simulink model "INFLW_2"  (R2022b)
settings: Solver=FixedStepDiscrete  StartTime=0  StopTime=duration  FixedStep=sample_time  RelTol=1e-3
values from neighbouring files (symbols this model uses):
  ParInflow =     [INFLW_2_params.mat]
  sample_time = 0.1    [INFLW_2_params.mat]
libraries: simulink x15, dspstat3 x11
settings Model: Creator=Carlo_TUM  LastModifiedBy=Carlo_TUM
settings DataIOCC: LoadExternalInput=on  ReturnWorkspaceOutputs=off  ReturnWorkspaceOutputsName=off
settings OptimizationCC: DefaultParameterBehavior=Inlined  EnhancedBackFolding=on  PassReuseOutputArgsAs=Individual arguments  OptimizeBlockOrder=speed  DifferentSizesBufferReuse=on  OptimizationCustomize=off  EfficientTunableParamExpr=on
settings DebuggingCC: ParameterTunabilityLossMsg=error
settings SFSimCC: MATLABDynamicMemAlloc=off
settings RTWCC: Description=Embedded Coder  SystemTargetFile=ert.tlc  TemplateMakefile=ert_default_tmf
settings CodeAppCC: ForceParamTrailComments=on  IgnoreCustomStorageClasses=off  OperatorAnnotations=on  SimulinkDataObjDesc=on  SFDataObjDesc=on  InsertBlockDesc=on
settings ERTTargetCC: TargetLangStandard=C99 (ISO)  GenerateSampleERTMain=on  InlinedParameterPlacement=NonHierarchical  ERTCustomFileTemplate=example_file_process.tlc

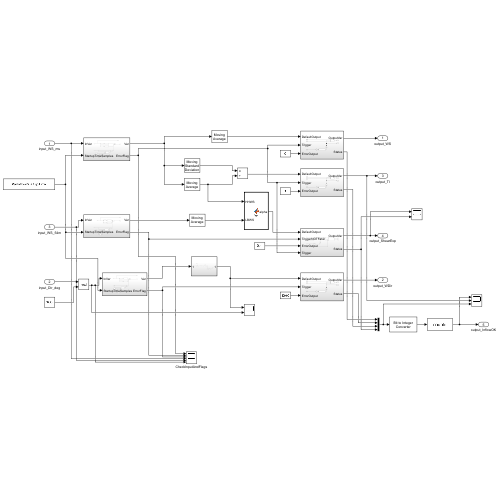
[thumbnail: Simulink's stored preview of the top-level diagram]
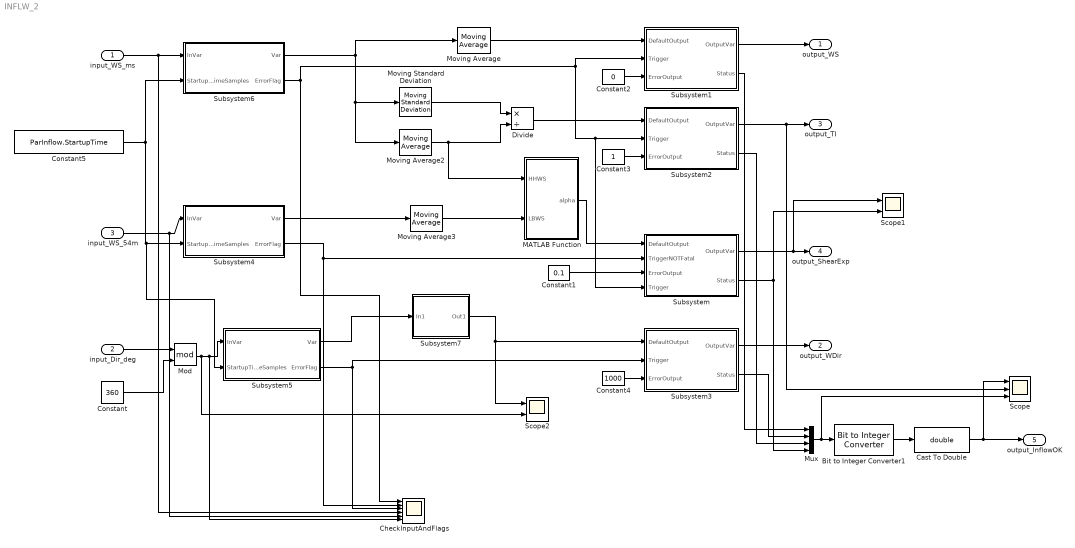
== system INFLW_2 ==
  input_WS_ms : Inport  PortDimensions=1
  input_Dir_deg : Inport  Port=2  PortDimensions=1
  input_WS_54m : Inport  Port=3  PortDimensions=1
  Bit to Integer Converter1 : simulink/Logic and Bit Operations/Bit to Integer Converter  nbits=4  bitOrder=MSB first  signedOutputValues=Unsigned  outDtype=Inherit via internal rule  outDtypeSigned=Inherit via internal rule
      settings: LibrarySourceBlock=|
      | commutil2/Bit to Integer
      | Converter
  Cast To Double : DataTypeConversion  OutDataTypeStr=double  SaturateOnIntegerOverflow=off  RndMeth=Floor
  CheckInputAndFlags : Scope  NumInputPorts=6
  Constant : Constant  Value=360
  Constant1 : Constant  Value=0.1
  Constant2 : Constant  Value=0
  Constant3 : Constant
  Constant4 : Constant  Value=1000
  Constant5 : Constant  Value=ParInflow.StartupTime
  Divide : Product  Inputs=*/
  MATLAB Function : MATLAB Function  TreatAsAtomicUnit=on
  Mod : Math  Operator=mod  SignedPower=on
  Moving Average : dspstat3/Moving Average  Method=Sliding window  ForgettingFactorPort=off  SpecifyWindowLength=on  WindowLength=ParInflow.MovAvWS  OverlapLength=ParInflow.MovAvWS -1  AllowArbitraryInputLength=off  ForgettingFactor=0.9  SimulateUsing=Code generation
  Moving Average2 : dspstat3/Moving Average  Method=Sliding window  ForgettingFactorPort=off  SpecifyWindowLength=on  WindowLength=ParInflow.MovAvTI  OverlapLength=ParInflow.MovAvTI - 1  AllowArbitraryInputLength=off  ForgettingFactor=0.9  SimulateUsing=Code generation
  Moving Average3 : dspstat3/Moving Average  Method=Sliding window  ForgettingFactorPort=off  SpecifyWindowLength=on  WindowLength=ParInflow.MovAvTI  OverlapLength=ParInflow.MovAvTI - 1  AllowArbitraryInputLength=off  ForgettingFactor=0.9  SimulateUsing=Code generation
  Moving Standard Deviation : dspstat3/Moving Standard Deviation  Method=Sliding window  ForgettingFactorPort=off  SpecifyWindowLength=on  WindowLength=ParInflow.MovAvTI  OverlapLength=ParInflow.MovAvTI - 1  AllowArbitraryInputLength=off  ForgettingFactor=0.9  SimulateUsing=Code generation
  Mux : Mux
  Scope : Scope  NumInputPorts=3
  Scope1 : Scope  NumInputPorts=2
  Scope2 : Scope  NumInputPorts=2
  Subsystem : Subsystem
  Subsystem1 : Subsystem
  Subsystem2 : Subsystem
  Subsystem3 : Subsystem
  Subsystem4 : Subsystem
  Subsystem5 : Subsystem
  Subsystem6 : Subsystem
  Subsystem7 : Subsystem
  output_WS : Outport  VectorParamsAs1DForOutWhenUnconnected=off
  output_WDir : Outport  Port=2  VectorParamsAs1DForOutWhenUnconnected=off
  output_TI : Outport  Port=3  VectorParamsAs1DForOutWhenUnconnected=off
  output_ShearExp : Outport  Port=4  VectorParamsAs1DForOutWhenUnconnected=off
  output_InflowOK : Outport  Port=5  VectorParamsAs1DForOutWhenUnconnected=off
  wires:
  Subsystem5/2(ErrorFlag) -> CheckInputAndFlags/3, Subsystem3/2(Trigger)
  Constant1/1 -> Subsystem/3(ErrorOutput)
  Subsystem5/1(Var) -> Subsystem7/1(In1)
  Constant4/1 -> Subsystem3/3(ErrorOutput)
  input_WS_ms/1 -> CheckInputAndFlags/4, Subsystem6/1(InVar)
  Bit to Integer Converter1/1 -> Cast To Double/1
  Constant5/1 -> Subsystem5/2(StartupTimeSamples), Subsystem4/2(StartupTimeSamples), Subsystem6/2(StartupTimeSamples)
  Cast To Double/1 -> Scope/1, output_InflowOK/1
  Constant2/1 -> Subsystem1/3(ErrorOutput)
  Constant/1 -> Mod/2
  Mod/1 -> Scope2/2, Subsystem5/1(InVar), CheckInputAndFlags/6
  Subsystem/1(OutputVar) -> Scope1/1, output_ShearExp/1
  Subsystem2/2(Status) -> Mux/3
  Subsystem6/1(Var) -> Moving Average/1, Moving Average2/1, Moving Standard Deviation/1
  Subsystem/2(Status) -> Scope1/2, Mux/4
  Subsystem7/1(Out1) -> Scope2/1, Subsystem3/1(DefaultOutput)
  input_WS_54m/1 -> CheckInputAndFlags/5, Subsystem4/1(InVar)
  Subsystem1/2(Status) -> Mux/1
  input_Dir_deg/1 -> Mod/1
  Moving Average3/1 -> MATLAB Function/2(LBWS)
  Subsystem4/1(Var) -> Moving Average3/1
  Moving Average2/1 -> MATLAB Function/1(HHWS), Divide/2
  Moving Standard Deviation/1 -> Divide/1
  Constant3/1 -> Subsystem2/3(ErrorOutput)
  Moving Average/1 -> Subsystem1/1(DefaultOutput)
  Subsystem6/2(ErrorFlag) -> Subsystem1/2(Trigger), Subsystem/4(Trigger), Subsystem2/2(Trigger), CheckInputAndFlags/1
  Subsystem3/2(Status) -> Mux/2
  MATLAB Function/1(alpha) -> Subsystem/1(DefaultOutput)
  Subsystem1/1(OutputVar) -> output_WS/1
  Divide/1 -> Subsystem2/1(DefaultOutput)
  Subsystem3/1(OutputVar) -> output_WDir/1
  Subsystem2/1(OutputVar) -> Scope/2, output_TI/1
  Subsystem4/2(ErrorFlag) -> Subsystem/2(TriggerNOTFatal), CheckInputAndFlags/2
  Mux/1 -> Scope/3, Bit to Integer Converter1/1

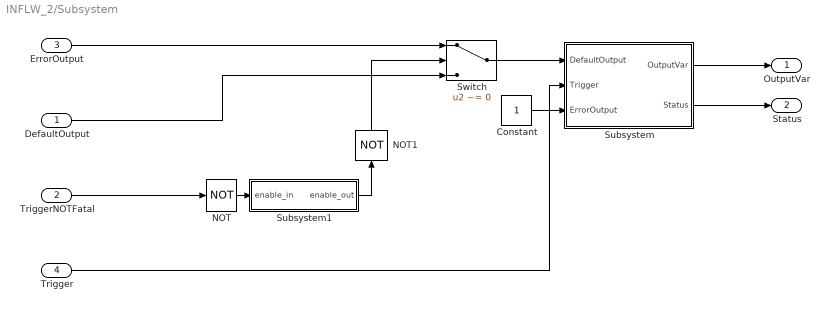
== system INFLW_2/Subsystem ==
  DefaultOutput : Inport
  TriggerNOTFatal : Inport  Port=2
  ErrorOutput : Inport  Port=3
  Trigger : Inport  Port=4
  Constant : Constant
  NOT : Logic  Operator=NOT  IconShape=distinctive  AllPortsSameDT=off  OutDataTypeStr=boolean
  NOT1 : Logic  Operator=NOT  IconShape=distinctive  AllPortsSameDT=off  OutDataTypeStr=boolean
  Subsystem : Subsystem
  Subsystem1 : Subsystem  mask(Signal holding){wait_time=ParInflow.ErrorChecks_WaitTime, sampling_time=sample_time, selection=on}
      mask prompts: wait_time "Wait time [s]"; sampling_time "Sampling time [s]"; selection "Instant disabling"
      mask help:
      | The block prevents fast switching of the input signal. After the input is changed, it waits for the defined time before changing the output, if the input doesn't change within this period, the output is switched.
      | The option "Instant disabling" only enforces waiting time on rising edge, but always allows the signal to go to zero.
      | Ask Vlaho for help.
      mask init:
      | Counter = wait_time/sampling_time;
      mask Help:
      | No documentation, ask Vlaho for help. ;)
      | 22 Nov 2020
  Switch : Switch  Criteria=u2 ~= 0  SaturateOnIntegerOverflow=off  InputSameDT=off
  OutputVar : Outport  VectorParamsAs1DForOutWhenUnconnected=off
  Status : Outport  Port=2  VectorParamsAs1DForOutWhenUnconnected=off
  wires:
  NOT1/1 -> Switch/2
  ErrorOutput/1 -> Switch/1
  Switch/1 -> Subsystem/1(DefaultOutput)
  DefaultOutput/1 -> Switch/3
  NOT/1 -> Subsystem1/1(enable_in)
  Subsystem1/1(enable_out) -> NOT1/1
  TriggerNOTFatal/1 -> NOT/1
  Subsystem/1(OutputVar) -> OutputVar/1
  Trigger/1 -> Subsystem/2(Trigger)
  Subsystem/2(Status) -> Status/1
  Constant/1 -> Subsystem/3(ErrorOutput)

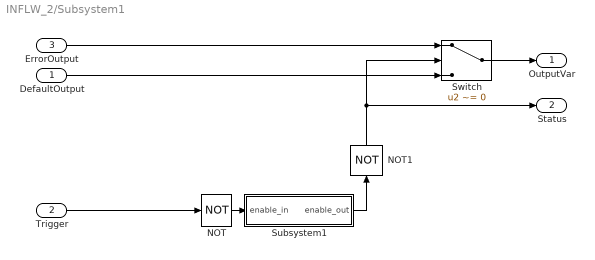
== system INFLW_2/Subsystem1 ==
  DefaultOutput : Inport
  Trigger : Inport  Port=2
  ErrorOutput : Inport  Port=3
  NOT : Logic  Operator=NOT  IconShape=distinctive  AllPortsSameDT=off  OutDataTypeStr=boolean
  NOT1 : Logic  Operator=NOT  IconShape=distinctive  AllPortsSameDT=off  OutDataTypeStr=boolean
  Subsystem1 : Subsystem  mask(Signal holding){wait_time=ParInflow.ErrorChecks_WaitTime, sampling_time=sample_time, selection=on}
      mask prompts: wait_time "Wait time [s]"; sampling_time "Sampling time [s]"; selection "Instant disabling"
      mask help:
      | The block prevents fast switching of the input signal. After the input is changed, it waits for the defined time before changing the output, if the input doesn't change within this period, the output is switched.
      | The option "Instant disabling" only enforces waiting time on rising edge, but always allows the signal to go to zero.
      | Ask Vlaho for help.
      mask init:
      | Counter = wait_time/sampling_time;
      mask Help:
      | No documentation, ask Vlaho for help. ;)
      | 22 Nov 2020
  Switch : Switch  Criteria=u2 ~= 0  SaturateOnIntegerOverflow=off  InputSameDT=off
  OutputVar : Outport  VectorParamsAs1DForOutWhenUnconnected=off
  Status : Outport  Port=2  VectorParamsAs1DForOutWhenUnconnected=off
  wires:
  Trigger/1 -> NOT/1
  Subsystem1/1(enable_out) -> NOT1/1
  NOT/1 -> Subsystem1/1(enable_in)
  DefaultOutput/1 -> Switch/3
  Switch/1 -> OutputVar/1
  ErrorOutput/1 -> Switch/1
  NOT1/1 -> Status/1, Switch/2

== system INFLW_2/Subsystem2 ==
  DefaultOutput : Inport
  Trigger : Inport  Port=2
  ErrorOutput : Inport  Port=3
  NOT : Logic  Operator=NOT  IconShape=distinctive  AllPortsSameDT=off  OutDataTypeStr=boolean
  NOT1 : Logic  Operator=NOT  IconShape=distinctive  AllPortsSameDT=off  OutDataTypeStr=boolean
  Subsystem1 : Subsystem  mask(Signal holding){wait_time=ParInflow.ErrorChecks_WaitTime, sampling_time=sample_time, selection=on}
      mask prompts: wait_time "Wait time [s]"; sampling_time "Sampling time [s]"; selection "Instant disabling"
      mask help:
      | The block prevents fast switching of the input signal. After the input is changed, it waits for the defined time before changing the output, if the input doesn't change within this period, the output is switched.
      | The option "Instant disabling" only enforces waiting time on rising edge, but always allows the signal to go to zero.
      | Ask Vlaho for help.
      mask init:
      | Counter = wait_time/sampling_time;
      mask Help:
      | No documentation, ask Vlaho for help. ;)
      | 22 Nov 2020
  Switch : Switch  Criteria=u2 ~= 0  SaturateOnIntegerOverflow=off  InputSameDT=off
  OutputVar : Outport  VectorParamsAs1DForOutWhenUnconnected=off
  Status : Outport  Port=2  VectorParamsAs1DForOutWhenUnconnected=off
  wires:
  NOT1/1 -> Switch/2, Status/1
  ErrorOutput/1 -> Switch/1
  Switch/1 -> OutputVar/1
  DefaultOutput/1 -> Switch/3
  NOT/1 -> Subsystem1/1(enable_in)
  Subsystem1/1(enable_out) -> NOT1/1
  Trigger/1 -> NOT/1

== system INFLW_2/Subsystem3 ==
  DefaultOutput : Inport
  Trigger : Inport  Port=2
  ErrorOutput : Inport  Port=3
  NOT : Logic  Operator=NOT  IconShape=distinctive  AllPortsSameDT=off  OutDataTypeStr=boolean
  NOT1 : Logic  Operator=NOT  IconShape=distinctive  AllPortsSameDT=off  OutDataTypeStr=boolean
  Subsystem1 : Subsystem  mask(Signal holding){wait_time=ParInflow.ErrorChecks_WaitTime, sampling_time=sample_time, selection=on}
      mask prompts: wait_time "Wait time [s]"; sampling_time "Sampling time [s]"; selection "Instant disabling"
      mask help:
      | The block prevents fast switching of the input signal. After the input is changed, it waits for the defined time before changing the output, if the input doesn't change within this period, the output is switched.
      | The option "Instant disabling" only enforces waiting time on rising edge, but always allows the signal to go to zero.
      | Ask Vlaho for help.
      mask init:
      | Counter = wait_time/sampling_time;
      mask Help:
      | No documentation, ask Vlaho for help. ;)
      | 22 Nov 2020
  Switch : Switch  Criteria=u2 ~= 0  SaturateOnIntegerOverflow=off  InputSameDT=off
  OutputVar : Outport  VectorParamsAs1DForOutWhenUnconnected=off
  Status : Outport  Port=2  VectorParamsAs1DForOutWhenUnconnected=off
  wires:
  Trigger/1 -> NOT/1
  Subsystem1/1(enable_out) -> NOT1/1
  NOT/1 -> Subsystem1/1(enable_in)
  DefaultOutput/1 -> Switch/3
  Switch/1 -> OutputVar/1
  ErrorOutput/1 -> Switch/1
  NOT1/1 -> Status/1, Switch/2

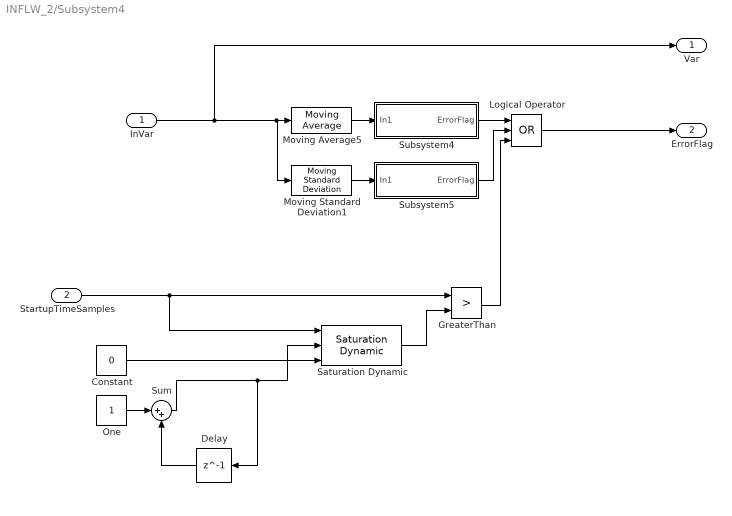
== system INFLW_2/Subsystem4 ==
  InVar : Inport
  StartupTimeSamples : Inport  Port=2
  Constant : Constant  Value=0
  Delay : Delay  DelayLength=1  InitialCondition=0
  GreaterThan : RelationalOperator  Operator=>  OutDataTypeStr=boolean  RndMeth=Simplest  InputSameDT=off
  Logical Operator : Logic  Operator=OR  Inputs=3  AllPortsSameDT=off  OutDataTypeStr=boolean
  Moving Average5 : dspstat3/Moving Average  Method=Sliding window  ForgettingFactorPort=off  SpecifyWindowLength=on  WindowLength=ParInflow.MovAvErrorCheck  OverlapLength=ParInflow.MovAvErrorCheck - 1  AllowArbitraryInputLength=off  ForgettingFactor=0.9  SimulateUsing=Code generation
  Moving Standard Deviation1 : dspstat3/Moving Standard Deviation  Method=Sliding window  ForgettingFactorPort=off  SpecifyWindowLength=on  WindowLength=ParInflow.MovAvErrorCheck  OverlapLength=ParInflow.MovAvErrorCheck - 1  AllowArbitraryInputLength=off  ForgettingFactor=0.9  SimulateUsing=Code generation
  One : Constant  OutDataTypeStr=Inherit: Inherit via back propagation
  Saturation Dynamic : simulink/Discontinuities/Saturation Dynamic  OutMin=[]  OutMax=[]  OutDataTypeStr=Inherit: Same as second input  OutDataType=fixdt(1, 16)  OutScaling=2^-10  DoSatur=off
  Subsystem4 : Subsystem
  Subsystem5 : Subsystem
  Sum : Sum  Inputs=|++
  Var : Outport  VectorParamsAs1DForOutWhenUnconnected=off
  ErrorFlag : Outport  Port=2  VectorParamsAs1DForOutWhenUnconnected=off
  wires:
  Logical Operator/1 -> ErrorFlag/1
  Subsystem5/1(ErrorFlag) -> Logical Operator/2
  Moving Standard Deviation1/1 -> Subsystem5/1(In1)
  Subsystem4/1(ErrorFlag) -> Logical Operator/1
  Moving Average5/1 -> Subsystem4/1(In1)
  InVar/1 -> Moving Average5/1, Moving Standard Deviation1/1, Var/1
  Constant/1 -> Saturation Dynamic/3
  Delay/1 -> Sum/2
  StartupTimeSamples/1 -> Saturation Dynamic/1, GreaterThan/1
  GreaterThan/1 -> Logical Operator/3
  Saturation Dynamic/1 -> GreaterThan/2
  Sum/1 -> Delay/1, Saturation Dynamic/2
  One/1 -> Sum/1

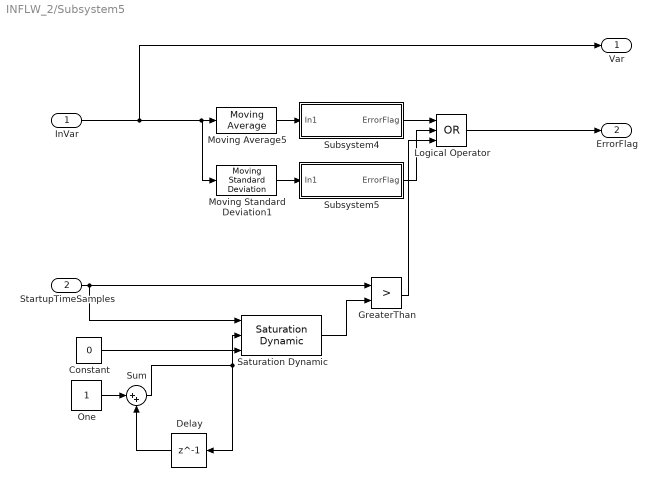
== system INFLW_2/Subsystem5 ==
  InVar : Inport
  StartupTimeSamples : Inport  Port=2
  Constant : Constant  Value=0
  Delay : Delay  DelayLength=1  InitialCondition=0
  GreaterThan : RelationalOperator  Operator=>  OutDataTypeStr=boolean  RndMeth=Simplest  InputSameDT=off
  Logical Operator : Logic  Operator=OR  Inputs=3  AllPortsSameDT=off  OutDataTypeStr=boolean
  Moving Average5 : dspstat3/Moving Average  Method=Sliding window  ForgettingFactorPort=off  SpecifyWindowLength=on  WindowLength=ParInflow.MovAvErrorCheck  OverlapLength=ParInflow.MovAvErrorCheck - 1  AllowArbitraryInputLength=off  ForgettingFactor=0.9  SimulateUsing=Code generation
  Moving Standard Deviation1 : dspstat3/Moving Standard Deviation  Method=Sliding window  ForgettingFactorPort=off  SpecifyWindowLength=on  WindowLength=ParInflow.MovAvErrorCheck  OverlapLength=ParInflow.MovAvErrorCheck - 1  AllowArbitraryInputLength=off  ForgettingFactor=0.9  SimulateUsing=Code generation
  One : Constant  OutDataTypeStr=Inherit: Inherit via back propagation
  Saturation Dynamic : simulink/Discontinuities/Saturation Dynamic  OutMin=[]  OutMax=[]  OutDataTypeStr=Inherit: Same as second input  OutDataType=fixdt(1, 16)  OutScaling=2^-10  DoSatur=off
  Subsystem4 : Subsystem
  Subsystem5 : Subsystem
  Sum : Sum  Inputs=|++
  Var : Outport  VectorParamsAs1DForOutWhenUnconnected=off
  ErrorFlag : Outport  Port=2  VectorParamsAs1DForOutWhenUnconnected=off
  wires:
  InVar/1 -> Var/1, Moving Standard Deviation1/1, Moving Average5/1
  Moving Average5/1 -> Subsystem4/1(In1)
  Subsystem4/1(ErrorFlag) -> Logical Operator/1
  Moving Standard Deviation1/1 -> Subsystem5/1(In1)
  Subsystem5/1(ErrorFlag) -> Logical Operator/2
  Logical Operator/1 -> ErrorFlag/1
  Constant/1 -> Saturation Dynamic/3
  Delay/1 -> Sum/2
  StartupTimeSamples/1 -> Saturation Dynamic/1, GreaterThan/1
  GreaterThan/1 -> Logical Operator/3
  Saturation Dynamic/1 -> GreaterThan/2
  Sum/1 -> Delay/1, Saturation Dynamic/2
  One/1 -> Sum/1

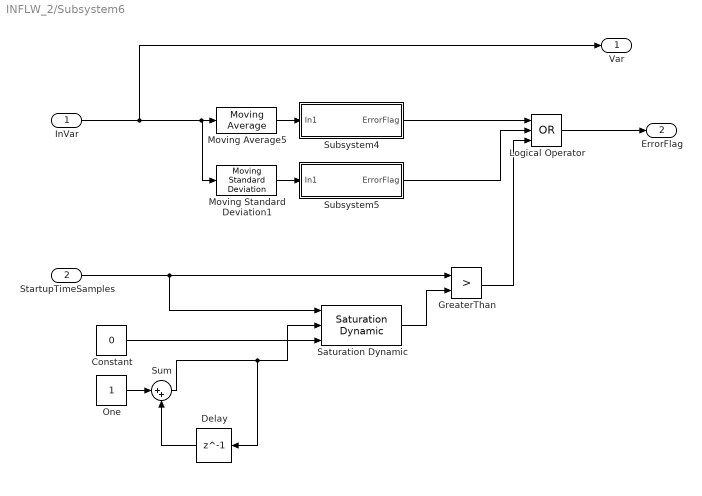
== system INFLW_2/Subsystem6 ==
  InVar : Inport
  StartupTimeSamples : Inport  Port=2
  Constant : Constant  Value=0
  Delay : Delay  DelayLength=1  InitialCondition=0
  GreaterThan : RelationalOperator  Operator=>  OutDataTypeStr=boolean  RndMeth=Simplest  InputSameDT=off
  Logical Operator : Logic  Operator=OR  Inputs=3  AllPortsSameDT=off  OutDataTypeStr=boolean
  Moving Average5 : dspstat3/Moving Average  Method=Sliding window  ForgettingFactorPort=off  SpecifyWindowLength=on  WindowLength=ParInflow.MovAvErrorCheck  OverlapLength=ParInflow.MovAvErrorCheck - 1  AllowArbitraryInputLength=off  ForgettingFactor=0.9  SimulateUsing=Code generation
  Moving Standard Deviation1 : dspstat3/Moving Standard Deviation  Method=Sliding window  ForgettingFactorPort=off  SpecifyWindowLength=on  WindowLength=ParInflow.MovAvErrorCheck  OverlapLength=ParInflow.MovAvErrorCheck -1  AllowArbitraryInputLength=off  ForgettingFactor=0.9  SimulateUsing=Code generation
  One : Constant  OutDataTypeStr=Inherit: Inherit via back propagation
  Saturation Dynamic : simulink/Discontinuities/Saturation Dynamic  OutMin=[]  OutMax=[]  OutDataTypeStr=Inherit: Same as second input  OutDataType=fixdt(1, 16)  OutScaling=2^-10  DoSatur=off
  Subsystem4 : Subsystem
  Subsystem5 : Subsystem
  Sum : Sum  Inputs=|++
  Var : Outport  VectorParamsAs1DForOutWhenUnconnected=off
  ErrorFlag : Outport  Port=2  VectorParamsAs1DForOutWhenUnconnected=off
  wires:
  InVar/1 -> Var/1, Moving Standard Deviation1/1, Moving Average5/1
  Moving Average5/1 -> Subsystem4/1(In1)
  Subsystem4/1(ErrorFlag) -> Logical Operator/1
  Moving Standard Deviation1/1 -> Subsystem5/1(In1)
  Subsystem5/1(ErrorFlag) -> Logical Operator/2
  Logical Operator/1 -> ErrorFlag/1
  StartupTimeSamples/1 -> Saturation Dynamic/1, GreaterThan/1
  Sum/1 -> Delay/1, Saturation Dynamic/2
  One/1 -> Sum/1
  Delay/1 -> Sum/2
  GreaterThan/1 -> Logical Operator/3
  Constant/1 -> Saturation Dynamic/3
  Saturation Dynamic/1 -> GreaterThan/2

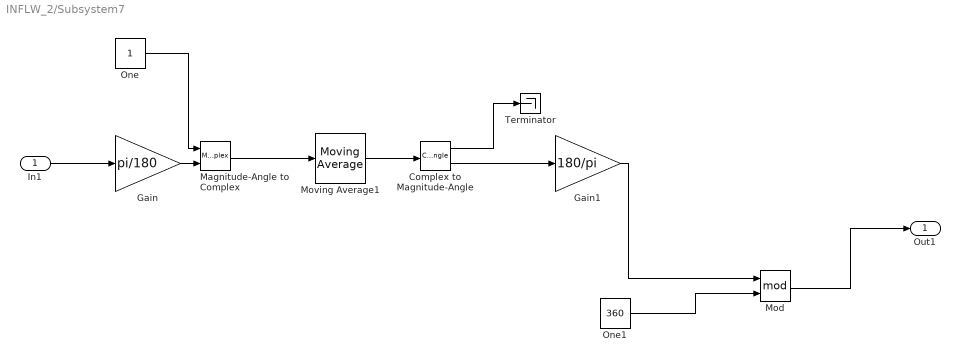
== system INFLW_2/Subsystem7 ==
  In1 : Inport
  Complex to Magnitude-Angle : ComplexToMagnitudeAngle
  Gain : Gain  Gain=pi/180
  Gain1 : Gain  Gain=180/pi
  Magnitude-Angle to Complex : MagnitudeAngleToComplex
  Mod : Math  Operator=mod  SignedPower=on
  Moving Average1 : dspstat3/Moving Average  Method=Sliding window  ForgettingFactorPort=off  SpecifyWindowLength=on  WindowLength=ParInflow.MovAvWDir  OverlapLength=ParInflow.MovAvWDir - 1  AllowArbitraryInputLength=off  ForgettingFactor=0.9  SimulateUsing=Code generation
  One : Constant  OutDataTypeStr=Inherit: Inherit via back propagation
  One1 : Constant  Value=360  OutDataTypeStr=Inherit: Inherit via back propagation
  Terminator : Terminator
  Out1 : Outport  VectorParamsAs1DForOutWhenUnconnected=off
  wires:
  Complex to Magnitude-Angle/2 -> Gain1/1
  In1/1 -> Gain/1
  One/1 -> Magnitude-Angle to Complex/1
  Gain/1 -> Magnitude-Angle to Complex/2
  Magnitude-Angle to Complex/1 -> Moving Average1/1
  Moving Average1/1 -> Complex to Magnitude-Angle/1
  Complex to Magnitude-Angle/1 -> Terminator/1
  Gain1/1 -> Mod/1
  One1/1 -> Mod/2
  Mod/1 -> Out1/1

== system INFLW_2/Subsystem/Subsystem ==
  DefaultOutput : Inport
  Trigger : Inport  Port=2
  ErrorOutput : Inport  Port=3
  NOT : Logic  Operator=NOT  IconShape=distinctive  AllPortsSameDT=off  OutDataTypeStr=boolean
  NOT1 : Logic  Operator=NOT  IconShape=distinctive  AllPortsSameDT=off  OutDataTypeStr=boolean
  Subsystem1 : Subsystem  mask(Signal holding){wait_time=ParInflow.ErrorChecks_WaitTime, sampling_time=sample_time, selection=on}
      mask prompts: wait_time "Wait time [s]"; sampling_time "Sampling time [s]"; selection "Instant disabling"
      mask help:
      | The block prevents fast switching of the input signal. After the input is changed, it waits for the defined time before changing the output, if the input doesn't change within this period, the output is switched.
      | The option "Instant disabling" only enforces waiting time on rising edge, but always allows the signal to go to zero.
      | Ask Vlaho for help.
      mask init:
      | Counter = wait_time/sampling_time;
      mask Help:
      | No documentation, ask Vlaho for help. ;)
      | 22 Nov 2020
  Switch : Switch  Criteria=u2 ~= 0  SaturateOnIntegerOverflow=off  InputSameDT=off
  OutputVar : Outport  VectorParamsAs1DForOutWhenUnconnected=off
  Status : Outport  Port=2  VectorParamsAs1DForOutWhenUnconnected=off
  wires:
  NOT1/1 -> Switch/2, Status/1
  ErrorOutput/1 -> Switch/1
  Switch/1 -> OutputVar/1
  DefaultOutput/1 -> Switch/3
  NOT/1 -> Subsystem1/1(enable_in)
  Subsystem1/1(enable_out) -> NOT1/1
  Trigger/1 -> NOT/1

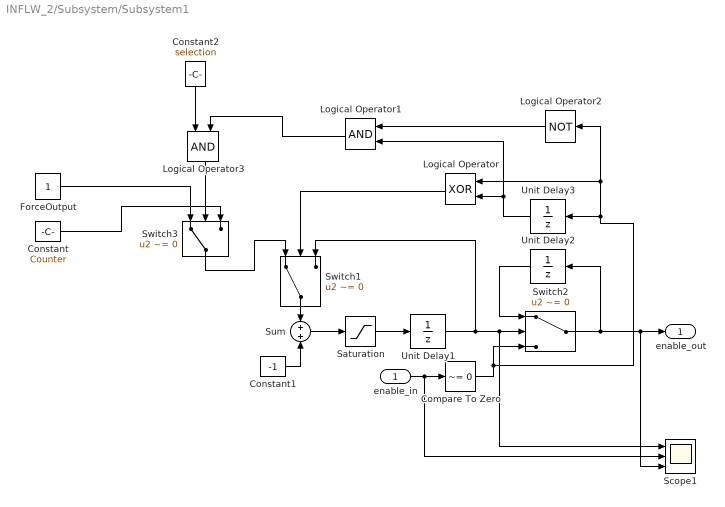
== system INFLW_2/Subsystem/Subsystem1 ==
  enable_in : Inport
  Compare To Zero : simulink/Logic and Bit Operations/Compare To Zero  relop=~=  OutDataTypeStr=boolean
  Constant : Constant  Value=Counter
  Constant1 : Constant  Value=-1
  Constant2 : Constant  Value=selection
  ForceOutput : Constant  OutDataTypeStr=Inherit: Inherit via back propagation
  Logical Operator : Logic  Operator=XOR  AllPortsSameDT=off  OutDataTypeStr=boolean
  Logical Operator1 : Logic  AllPortsSameDT=off  OutDataTypeStr=boolean
  Logical Operator2 : Logic  Operator=NOT  AllPortsSameDT=off  OutDataTypeStr=boolean
  Logical Operator3 : Logic  AllPortsSameDT=off  OutDataTypeStr=boolean
  Saturation : Saturate  UpperLimit=inf  LowerLimit=-inf
  Scope1 : Scope  NumInputPorts=3
  Sum : Sum
  Switch1 : Switch  Criteria=u2 ~= 0  SaturateOnIntegerOverflow=off  InputSameDT=off
  Switch2 : Switch  Criteria=u2 ~= 0  SaturateOnIntegerOverflow=off  InputSameDT=off
  Switch3 : Switch  Criteria=u2 ~= 0  SaturateOnIntegerOverflow=off  InputSameDT=off
  Unit Delay1 : UnitDelay  SampleTime=sampling_time  HasFrameUpgradeWarning=on
  Unit Delay2 : UnitDelay  SampleTime=sampling_time  HasFrameUpgradeWarning=on
  Unit Delay3 : UnitDelay  SampleTime=sampling_time  HasFrameUpgradeWarning=on
  enable_out : Outport
  wires:
  Saturation/1 -> Unit Delay1/1
  Unit Delay2/1 -> Switch2/1
  Switch2/1 -> Scope1/3, enable_out/1, Unit Delay2/1
  Sum/1 -> Saturation/1
  Switch1/1 -> Sum/1
  Constant1/1 -> Sum/2
  Constant/1 -> Switch3/3
  Logical Operator/1 -> Switch1/2
  enable_in/1 -> Scope1/2, Compare To Zero/1
  Logical Operator2/1 -> Logical Operator1/1
  Logical Operator1/1 -> Logical Operator3/2
  Compare To Zero/1 -> Switch2/3, Unit Delay3/1, Logical Operator/1, Logical Operator2/1
  Unit Delay3/1 -> Logical Operator/2, Logical Operator1/2
  Unit Delay1/1 -> Switch1/3, Scope1/1, Switch2/2
  Constant2/1 -> Logical Operator3/1
  ForceOutput/1 -> Switch3/1
  Switch3/1 -> Switch1/1
  Logical Operator3/1 -> Switch3/2

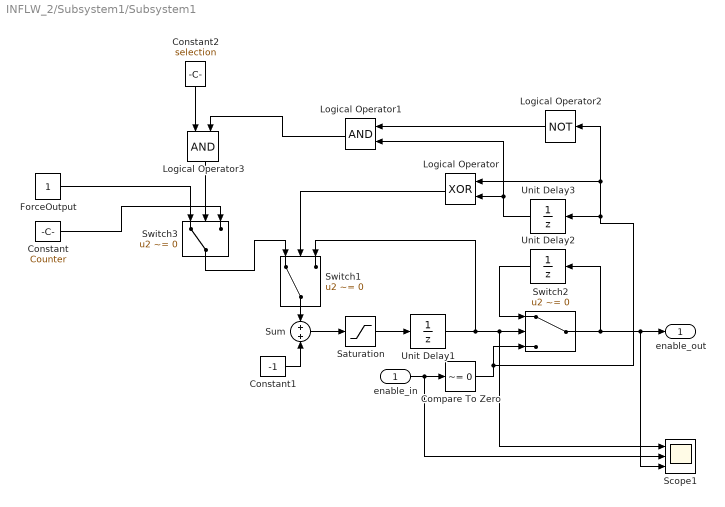
== system INFLW_2/Subsystem1/Subsystem1 ==
  enable_in : Inport
  Compare To Zero : simulink/Logic and Bit Operations/Compare To Zero  relop=~=  OutDataTypeStr=boolean
  Constant : Constant  Value=Counter
  Constant1 : Constant  Value=-1
  Constant2 : Constant  Value=selection
  ForceOutput : Constant  OutDataTypeStr=Inherit: Inherit via back propagation
  Logical Operator : Logic  Operator=XOR  AllPortsSameDT=off  OutDataTypeStr=boolean
  Logical Operator1 : Logic  AllPortsSameDT=off  OutDataTypeStr=boolean
  Logical Operator2 : Logic  Operator=NOT  AllPortsSameDT=off  OutDataTypeStr=boolean
  Logical Operator3 : Logic  AllPortsSameDT=off  OutDataTypeStr=boolean
  Saturation : Saturate  UpperLimit=inf  LowerLimit=-inf
  Scope1 : Scope  NumInputPorts=3
  Sum : Sum
  Switch1 : Switch  Criteria=u2 ~= 0  SaturateOnIntegerOverflow=off  InputSameDT=off
  Switch2 : Switch  Criteria=u2 ~= 0  SaturateOnIntegerOverflow=off  InputSameDT=off
  Switch3 : Switch  Criteria=u2 ~= 0  SaturateOnIntegerOverflow=off  InputSameDT=off
  Unit Delay1 : UnitDelay  SampleTime=sampling_time  HasFrameUpgradeWarning=on
  Unit Delay2 : UnitDelay  SampleTime=sampling_time  HasFrameUpgradeWarning=on
  Unit Delay3 : UnitDelay  SampleTime=sampling_time  HasFrameUpgradeWarning=on
  enable_out : Outport
  wires:
  Logical Operator3/1 -> Switch3/2
  Switch3/1 -> Switch1/1
  ForceOutput/1 -> Switch3/1
  Constant2/1 -> Logical Operator3/1
  Unit Delay1/1 -> Switch2/2, Scope1/1, Switch1/3
  Unit Delay3/1 -> Logical Operator1/2, Logical Operator/2
  Compare To Zero/1 -> Logical Operator2/1, Logical Operator/1, Unit Delay3/1, Switch2/3
  Logical Operator1/1 -> Logical Operator3/2
  Logical Operator2/1 -> Logical Operator1/1
  enable_in/1 -> Compare To Zero/1, Scope1/2
  Logical Operator/1 -> Switch1/2
  Constant/1 -> Switch3/3
  Constant1/1 -> Sum/2
  Switch1/1 -> Sum/1
  Sum/1 -> Saturation/1
  Switch2/1 -> Unit Delay2/1, enable_out/1, Scope1/3
  Unit Delay2/1 -> Switch2/1
  Saturation/1 -> Unit Delay1/1

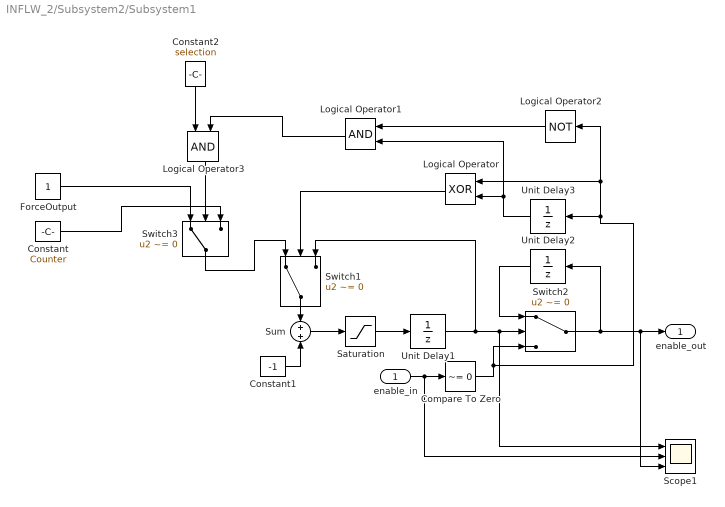
== system INFLW_2/Subsystem2/Subsystem1 ==
  enable_in : Inport
  Compare To Zero : simulink/Logic and Bit Operations/Compare To Zero  relop=~=  OutDataTypeStr=boolean
  Constant : Constant  Value=Counter
  Constant1 : Constant  Value=-1
  Constant2 : Constant  Value=selection
  ForceOutput : Constant  OutDataTypeStr=Inherit: Inherit via back propagation
  Logical Operator : Logic  Operator=XOR  AllPortsSameDT=off  OutDataTypeStr=boolean
  Logical Operator1 : Logic  AllPortsSameDT=off  OutDataTypeStr=boolean
  Logical Operator2 : Logic  Operator=NOT  AllPortsSameDT=off  OutDataTypeStr=boolean
  Logical Operator3 : Logic  AllPortsSameDT=off  OutDataTypeStr=boolean
  Saturation : Saturate  UpperLimit=inf  LowerLimit=-inf
  Scope1 : Scope  NumInputPorts=3
  Sum : Sum
  Switch1 : Switch  Criteria=u2 ~= 0  SaturateOnIntegerOverflow=off  InputSameDT=off
  Switch2 : Switch  Criteria=u2 ~= 0  SaturateOnIntegerOverflow=off  InputSameDT=off
  Switch3 : Switch  Criteria=u2 ~= 0  SaturateOnIntegerOverflow=off  InputSameDT=off
  Unit Delay1 : UnitDelay  SampleTime=sampling_time  HasFrameUpgradeWarning=on
  Unit Delay2 : UnitDelay  SampleTime=sampling_time  HasFrameUpgradeWarning=on
  Unit Delay3 : UnitDelay  SampleTime=sampling_time  HasFrameUpgradeWarning=on
  enable_out : Outport
  wires:
  Saturation/1 -> Unit Delay1/1
  Unit Delay2/1 -> Switch2/1
  Switch2/1 -> Scope1/3, enable_out/1, Unit Delay2/1
  Sum/1 -> Saturation/1
  Switch1/1 -> Sum/1
  Constant1/1 -> Sum/2
  Constant/1 -> Switch3/3
  Logical Operator/1 -> Switch1/2
  enable_in/1 -> Scope1/2, Compare To Zero/1
  Logical Operator2/1 -> Logical Operator1/1
  Logical Operator1/1 -> Logical Operator3/2
  Compare To Zero/1 -> Switch2/3, Unit Delay3/1, Logical Operator/1, Logical Operator2/1
  Unit Delay3/1 -> Logical Operator/2, Logical Operator1/2
  Unit Delay1/1 -> Switch1/3, Scope1/1, Switch2/2
  Constant2/1 -> Logical Operator3/1
  ForceOutput/1 -> Switch3/1
  Switch3/1 -> Switch1/1
  Logical Operator3/1 -> Switch3/2

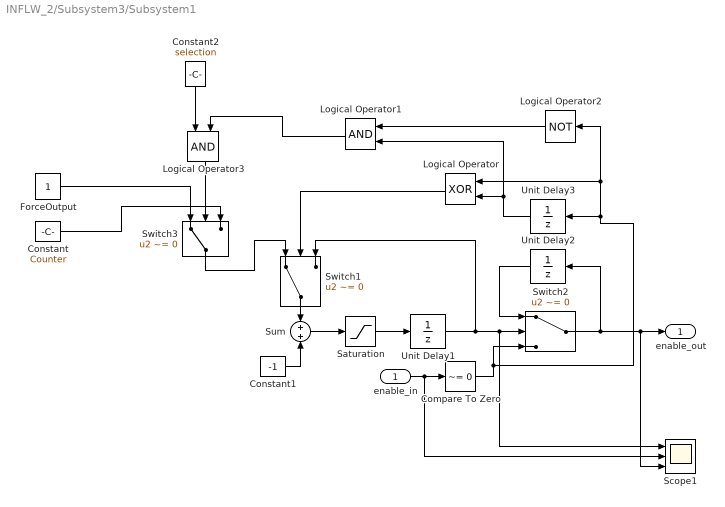
== system INFLW_2/Subsystem3/Subsystem1 ==
  enable_in : Inport
  Compare To Zero : simulink/Logic and Bit Operations/Compare To Zero  relop=~=  OutDataTypeStr=boolean
  Constant : Constant  Value=Counter
  Constant1 : Constant  Value=-1
  Constant2 : Constant  Value=selection
  ForceOutput : Constant  OutDataTypeStr=Inherit: Inherit via back propagation
  Logical Operator : Logic  Operator=XOR  AllPortsSameDT=off  OutDataTypeStr=boolean
  Logical Operator1 : Logic  AllPortsSameDT=off  OutDataTypeStr=boolean
  Logical Operator2 : Logic  Operator=NOT  AllPortsSameDT=off  OutDataTypeStr=boolean
  Logical Operator3 : Logic  AllPortsSameDT=off  OutDataTypeStr=boolean
  Saturation : Saturate  UpperLimit=inf  LowerLimit=-inf
  Scope1 : Scope  NumInputPorts=3
  Sum : Sum
  Switch1 : Switch  Criteria=u2 ~= 0  SaturateOnIntegerOverflow=off  InputSameDT=off
  Switch2 : Switch  Criteria=u2 ~= 0  SaturateOnIntegerOverflow=off  InputSameDT=off
  Switch3 : Switch  Criteria=u2 ~= 0  SaturateOnIntegerOverflow=off  InputSameDT=off
  Unit Delay1 : UnitDelay  SampleTime=sampling_time  HasFrameUpgradeWarning=on
  Unit Delay2 : UnitDelay  SampleTime=sampling_time  HasFrameUpgradeWarning=on
  Unit Delay3 : UnitDelay  SampleTime=sampling_time  HasFrameUpgradeWarning=on
  enable_out : Outport
  wires:
  Logical Operator3/1 -> Switch3/2
  Switch3/1 -> Switch1/1
  ForceOutput/1 -> Switch3/1
  Constant2/1 -> Logical Operator3/1
  Unit Delay1/1 -> Switch2/2, Scope1/1, Switch1/3
  Unit Delay3/1 -> Logical Operator1/2, Logical Operator/2
  Compare To Zero/1 -> Logical Operator2/1, Logical Operator/1, Unit Delay3/1, Switch2/3
  Logical Operator1/1 -> Logical Operator3/2
  Logical Operator2/1 -> Logical Operator1/1
  enable_in/1 -> Compare To Zero/1, Scope1/2
  Logical Operator/1 -> Switch1/2
  Constant/1 -> Switch3/3
  Constant1/1 -> Sum/2
  Switch1/1 -> Sum/1
  Sum/1 -> Saturation/1
  Switch2/1 -> Unit Delay2/1, enable_out/1, Scope1/3
  Unit Delay2/1 -> Switch2/1
  Saturation/1 -> Unit Delay1/1

== system INFLW_2/Subsystem4/Subsystem4 ==
  In1 : Inport
  Compare To Constant : simulink/Logic and Bit Operations/Compare To Constant  relop=<=  const=0.00001  OutDataTypeStr=boolean
  IsInf : RelationalOperator  Operator=isInf  OutDataTypeStr=boolean  RndMeth=Simplest  InputSameDT=off
  IsNaN : RelationalOperator  Operator=isNaN  OutDataTypeStr=boolean  RndMeth=Simplest  InputSameDT=off
  Logical Operator : Logic  Operator=OR  Inputs=3  AllPortsSameDT=off  OutDataTypeStr=boolean
  ErrorFlag : Outport  VectorParamsAs1DForOutWhenUnconnected=off
  wires:
  IsNaN/1 -> Logical Operator/2
  In1/1 -> Compare To Constant/1, IsNaN/1, IsInf/1
  IsInf/1 -> Logical Operator/3
  Logical Operator/1 -> ErrorFlag/1
  Compare To Constant/1 -> Logical Operator/1

== system INFLW_2/Subsystem4/Subsystem5 ==
  In1 : Inport
  Compare To Constant : simulink/Logic and Bit Operations/Compare To Constant  relop=<=  const=0.00001  OutDataTypeStr=boolean
  IsInf : RelationalOperator  Operator=isInf  OutDataTypeStr=boolean  RndMeth=Simplest  InputSameDT=off
  IsNaN : RelationalOperator  Operator=isNaN  OutDataTypeStr=boolean  RndMeth=Simplest  InputSameDT=off
  Logical Operator : Logic  Operator=OR  Inputs=3  AllPortsSameDT=off  OutDataTypeStr=boolean
  ErrorFlag : Outport  VectorParamsAs1DForOutWhenUnconnected=off
  wires:
  Compare To Constant/1 -> Logical Operator/1
  Logical Operator/1 -> ErrorFlag/1
  IsInf/1 -> Logical Operator/3
  In1/1 -> Compare To Constant/1, IsInf/1, IsNaN/1
  IsNaN/1 -> Logical Operator/2

== system INFLW_2/Subsystem5/Subsystem4 ==
  In1 : Inport
  Compare To Constant : simulink/Logic and Bit Operations/Compare To Constant  relop=<=  const=0.00001  OutDataTypeStr=boolean
  IsInf : RelationalOperator  Operator=isInf  OutDataTypeStr=boolean  RndMeth=Simplest  InputSameDT=off
  IsNaN : RelationalOperator  Operator=isNaN  OutDataTypeStr=boolean  RndMeth=Simplest  InputSameDT=off
  Logical Operator : Logic  Operator=OR  Inputs=3  AllPortsSameDT=off  OutDataTypeStr=boolean
  ErrorFlag : Outport  VectorParamsAs1DForOutWhenUnconnected=off
  wires:
  Compare To Constant/1 -> Logical Operator/1
  Logical Operator/1 -> ErrorFlag/1
  IsInf/1 -> Logical Operator/3
  In1/1 -> IsInf/1, IsNaN/1, Compare To Constant/1
  IsNaN/1 -> Logical Operator/2

== system INFLW_2/Subsystem5/Subsystem5 ==
  In1 : Inport
  Compare To Constant : simulink/Logic and Bit Operations/Compare To Constant  relop=<=  const=0.00001  OutDataTypeStr=boolean
  IsInf : RelationalOperator  Operator=isInf  OutDataTypeStr=boolean  RndMeth=Simplest  InputSameDT=off
  IsNaN : RelationalOperator  Operator=isNaN  OutDataTypeStr=boolean  RndMeth=Simplest  InputSameDT=off
  Logical Operator : Logic  Operator=OR  Inputs=3  AllPortsSameDT=off  OutDataTypeStr=boolean
  ErrorFlag : Outport  VectorParamsAs1DForOutWhenUnconnected=off
  wires:
  IsNaN/1 -> Logical Operator/2
  In1/1 -> IsNaN/1, IsInf/1, Compare To Constant/1
  IsInf/1 -> Logical Operator/3
  Logical Operator/1 -> ErrorFlag/1
  Compare To Constant/1 -> Logical Operator/1

== system INFLW_2/Subsystem6/Subsystem4 ==
  In1 : Inport
  Compare To Constant : simulink/Logic and Bit Operations/Compare To Constant  relop=<=  const=0.00001  OutDataTypeStr=boolean
  IsInf : RelationalOperator  Operator=isInf  OutDataTypeStr=boolean  RndMeth=Simplest  InputSameDT=off
  IsNaN : RelationalOperator  Operator=isNaN  OutDataTypeStr=boolean  RndMeth=Simplest  InputSameDT=off
  Logical Operator : Logic  Operator=OR  Inputs=3  AllPortsSameDT=off  OutDataTypeStr=boolean
  ErrorFlag : Outport  VectorParamsAs1DForOutWhenUnconnected=off
  wires:
  Compare To Constant/1 -> Logical Operator/1
  Logical Operator/1 -> ErrorFlag/1
  IsInf/1 -> Logical Operator/3
  In1/1 -> IsInf/1, IsNaN/1, Compare To Constant/1
  IsNaN/1 -> Logical Operator/2

== system INFLW_2/Subsystem6/Subsystem5 ==
  In1 : Inport
  Compare To Constant : simulink/Logic and Bit Operations/Compare To Constant  relop=<=  const=0.00001  OutDataTypeStr=boolean
  IsInf : RelationalOperator  Operator=isInf  OutDataTypeStr=boolean  RndMeth=Simplest  InputSameDT=off
  IsNaN : RelationalOperator  Operator=isNaN  OutDataTypeStr=boolean  RndMeth=Simplest  InputSameDT=off
  Logical Operator : Logic  Operator=OR  Inputs=3  AllPortsSameDT=off  OutDataTypeStr=boolean
  ErrorFlag : Outport  VectorParamsAs1DForOutWhenUnconnected=off
  wires:
  IsNaN/1 -> Logical Operator/2
  In1/1 -> IsNaN/1, IsInf/1, Compare To Constant/1
  IsInf/1 -> Logical Operator/3
  Logical Operator/1 -> ErrorFlag/1
  Compare To Constant/1 -> Logical Operator/1

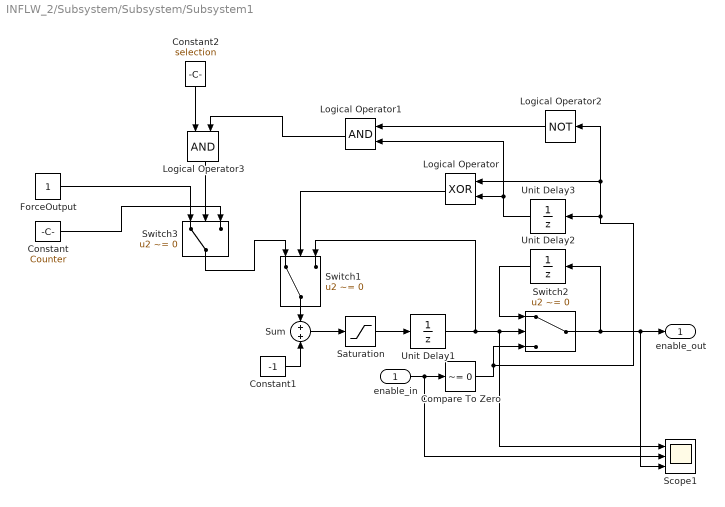
== system INFLW_2/Subsystem/Subsystem/Subsystem1 ==
  enable_in : Inport
  Compare To Zero : simulink/Logic and Bit Operations/Compare To Zero  relop=~=  OutDataTypeStr=boolean
  Constant : Constant  Value=Counter
  Constant1 : Constant  Value=-1
  Constant2 : Constant  Value=selection
  ForceOutput : Constant  OutDataTypeStr=Inherit: Inherit via back propagation
  Logical Operator : Logic  Operator=XOR  AllPortsSameDT=off  OutDataTypeStr=boolean
  Logical Operator1 : Logic  AllPortsSameDT=off  OutDataTypeStr=boolean
  Logical Operator2 : Logic  Operator=NOT  AllPortsSameDT=off  OutDataTypeStr=boolean
  Logical Operator3 : Logic  AllPortsSameDT=off  OutDataTypeStr=boolean
  Saturation : Saturate  UpperLimit=inf  LowerLimit=-inf
  Scope1 : Scope  NumInputPorts=3
  Sum : Sum
  Switch1 : Switch  Criteria=u2 ~= 0  SaturateOnIntegerOverflow=off  InputSameDT=off
  Switch2 : Switch  Criteria=u2 ~= 0  SaturateOnIntegerOverflow=off  InputSameDT=off
  Switch3 : Switch  Criteria=u2 ~= 0  SaturateOnIntegerOverflow=off  InputSameDT=off
  Unit Delay1 : UnitDelay  SampleTime=sampling_time  HasFrameUpgradeWarning=on
  Unit Delay2 : UnitDelay  SampleTime=sampling_time  HasFrameUpgradeWarning=on
  Unit Delay3 : UnitDelay  SampleTime=sampling_time  HasFrameUpgradeWarning=on
  enable_out : Outport
  wires:
  Saturation/1 -> Unit Delay1/1
  Unit Delay2/1 -> Switch2/1
  Switch2/1 -> Scope1/3, enable_out/1, Unit Delay2/1
  Sum/1 -> Saturation/1
  Switch1/1 -> Sum/1
  Constant1/1 -> Sum/2
  Constant/1 -> Switch3/3
  Logical Operator/1 -> Switch1/2
  enable_in/1 -> Scope1/2, Compare To Zero/1
  Logical Operator2/1 -> Logical Operator1/1
  Logical Operator1/1 -> Logical Operator3/2
  Compare To Zero/1 -> Switch2/3, Unit Delay3/1, Logical Operator/1, Logical Operator2/1
  Unit Delay3/1 -> Logical Operator/2, Logical Operator1/2
  Unit Delay1/1 -> Switch1/3, Scope1/1, Switch2/2
  Constant2/1 -> Logical Operator3/1
  ForceOutput/1 -> Switch3/1
  Switch3/1 -> Switch1/1
  Logical Operator3/1 -> Switch3/2

== matlab function INFLW_2/MATLAB Function ==
  data: HHWS input; alpha output; LBWS input
function alpha = fcn(HHWS, LBWS)

alpha = (log(HHWS) - log(LBWS))./(log(116.3) - log(54.2));
